simulink library "ServosLib"  (R2022b)
settings: Solver=VariableStepAuto  StartTime=0.0  StopTime=10.0  RelTol=1e-3
undefined symbols (not defined in the file): POS_hi, POS_lo, SimPar
libraries: simulink x2
settings Model: Creator=tbritton  LastModifiedBy=macheson
settings SolverCC: AlgebraicLoopSolver=TrustRegion
settings DebuggingCC: UnconnectedInputMsg=warning  UnconnectedOutputMsg=warning  UnconnectedLineMsg=warning  SFMachineParentedDataDiag=warning
settings ModelReferenceCC: EnableRefExpFcnMdlSchedulingChecks=on
settings RTWCC: DLArmComputeVersion=19.05

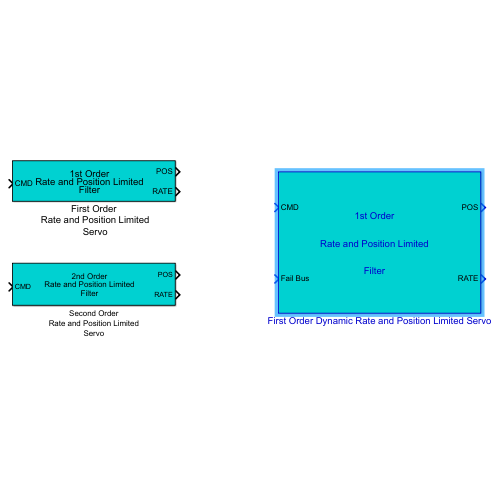
[thumbnail: Simulink's stored preview of the top-level diagram]
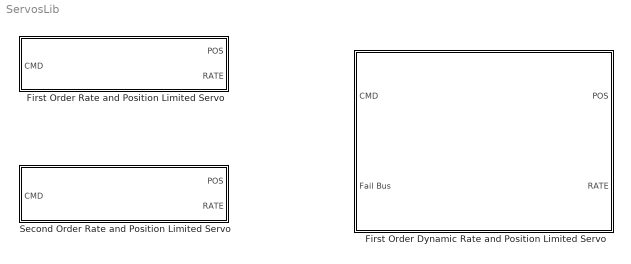
== system ServosLib ==
  First Order Rate and Position Limited Servo : Subsystem  mask(Rate and Position Limited Servo){freq=5, RL=300, POS_hi=30*pi/180, POS_lo=0*pi/180, Bias=0*pi/180, StateName=Actuators}
      mask prompts: freq "Bandwidth, Hz:"; RL "Rate Limit, rad/s:"; POS_hi "Position Limit High, rad:"; POS_lo "Position Limit Low, rad:"; Bias "Bias Value, rad:"; StateName "State Name:"
      mask help: First order transfer function: w/(s+w), with rate and position limits and output bias level.
      mask init:
      | %omega=2*pi*freq;
      mask Display:
      | text(.48,.70,'1st Order','horizontalAlignment','center');
      | text(.48,.50,'Rate and Position Limited','horizontalAlignment','center');
      | text(.48,.30,'Filter','horizontalAlignment','center');
  First Order Dynamic Rate and Position Limited Servo : Subsystem  mask(Rate and Position Limited Servo){freq=SimPar.Actuator.BW, Bias=SimPar.Actuator.Bias, StateName='Actuators'}
      mask prompts: freq "Bandwidth, Hz:"; Bias "Bias Value, rad:"; StateName "State Name:"
      mask help: First order transfer function: w/(s+w), with rate and position limits and output bias level.
      mask init:
      | %omega=2*pi*freq;
      mask Display:
      | text(.48,.70,'1st Order','horizontalAlignment','center');
      | text(.48,.50,'Rate and Position Limited','horizontalAlignment','center');
      | text(.48,.30,'Filter','horizontalAlignment','center');
  Second Order Rate and Position Limited Servo : Subsystem  mask(Rate and Position Limited Servo){freq=5, zeta=0.7, RL=300, POS_hi=30*pi/180, POS_lo=0*pi/180, Bias=0*pi/180, PosStateName=ActuatorPosition, RateStateName=ActuatorRate}
      mask prompts: freq "Bandwidth, Hz:"; zeta "Damping Ratio:"; RL "Rate Limit, rad/s:"; POS_hi "Position Limit High, rad:"; POS_lo "Position Limit Low, rad:"; Bias "Bias Value, rad:"; PosStateName "Position State Name:"; RateStateName "Rate State Name:"
      mask help: Second order transfer function: w^2/(s^2+2*zeta*w*s+w^2), with rate and position limits and output bias level.
      mask init:
      | %omega=2*pi*freq;
      mask Display:
      | text(.48,.70,'2nd Order','horizontalAlignment','center');
      | text(.48,.50,'Rate and Position Limited','horizontalAlignment','center');
      | text(.48,.30,'Filter','horizontalAlignment','center');

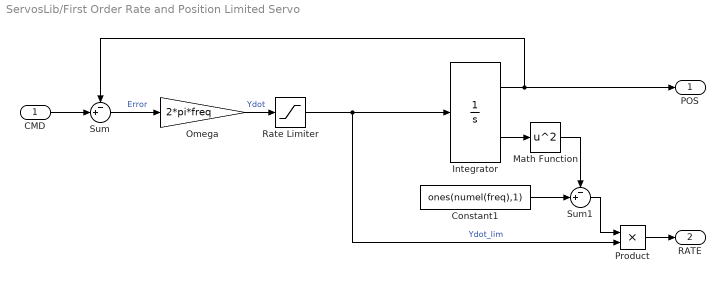
== system ServosLib/First Order Rate and Position Limited Servo ==
  CMD : Inport
  Constant1 : Constant  Value=ones(numel(freq),1)  VectorParams1D=off
  Integrator : Integrator  InitialCondition=Bias  LimitOutput=on  UpperSaturationLimit=POS_hi  LowerSaturationLimit=POS_lo  ShowSaturationPort=on  IgnoreLimit=on  ContinuousStateAttributes=StateName
  Math Function : Math  Operator=square  SignedPower=on
  Omega : Gain  Gain=2*pi*freq  SaturateOnIntegerOverflow=on  OutDataTypeStr=Inherit: Same as input  ParamDataTypeStr=Inherit: Same as input
  Product : Product  RndMeth=Zero
  Rate Limiter : Saturate  UpperLimit=RL  LowerLimit=-RL
  Sum : Sum  Inputs=-+|  InputSameDT=on  SaturateOnIntegerOverflow=on  OutDataTypeStr=Inherit: Same as first input
  Sum1 : Sum  Inputs=-+|  InputSameDT=on  SaturateOnIntegerOverflow=on  OutDataTypeStr=Inherit: Same as first input
  POS : Outport  VectorParamsAs1DForOutWhenUnconnected=off
  RATE : Outport  Port=2
  wires:
  CMD/1 -> Sum/2
  Rate Limiter/1 -> Integrator/1, Product/2  "Ydot_lim"
  Integrator/1 -> POS/1, Sum/1
  Sum/1 -> Omega/1  "Error"
  Omega/1 -> Rate Limiter/1  "Ydot"
  Integrator/2 -> Math Function/1
  Sum1/1 -> Product/1
  Product/1 -> RATE/1
  Constant1/1 -> Sum1/2
  Math Function/1 -> Sum1/1

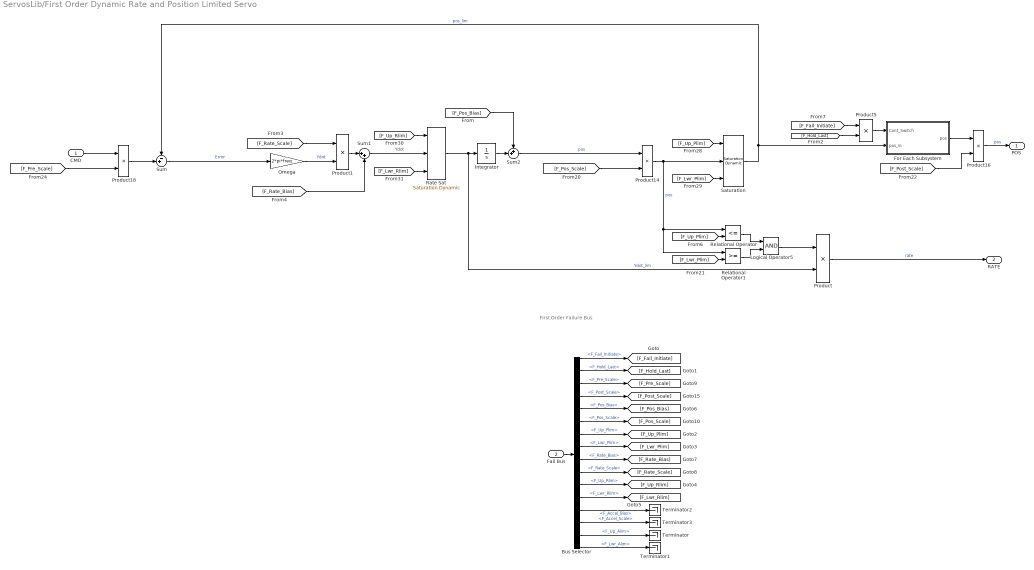
== system ServosLib/First Order Dynamic Rate and Position Limited Servo ==
  note: First Order Failure Bus
  CMD : Inport
  Fail Bus : Inport  Port=2
  Bus Selector : BusSelector  OutputSignals=F_Fail_Initiate,F_Hold_Last,F_Pre_Scale,F_Post_Scale,F_Pos_Bias,F_Pos_Scale,F_Up_Plim,F_Lwr_Plim,F_Rate_Bias,F_Rate_Scale,F_Up_Rlim,F_Lwr_Rlim,F_Accel_Bias,F_Accel_Scale,F_Up_Alim,F_Lwr_Alim
  For Each Subsystem : Subsystem  TreatAsAtomicUnit=on
  Integrator : Integrator  InitialCondition=Bias  UpperSaturationLimit=POS_hi  LowerSaturationLimit=POS_lo  IgnoreLimit=on  ContinuousStateAttributes=StateName
  Logical Operator5 : Logic  AllPortsSameDT=off  OutDataTypeStr=boolean
  Omega : Gain  Gain=2*pi*freq  SaturateOnIntegerOverflow=on  OutDataTypeStr=Inherit: Same as input  ParamDataTypeStr=Inherit: Same as input
  Product : Product  RndMeth=Zero
  Product{1,5,14,16,18} (5 alike) : Product
  Rate Sat : simulink/Discontinuities/Saturation Dynamic  OutMin=[]  OutMax=[]  OutDataTypeStr=Inherit: Same as second input  OutDataType=fixdt(1, 16)  OutScaling=2^-10  DoSatur=off
  Relational Operator : RelationalOperator  Operator=<=  OutDataTypeStr=boolean  RndMeth=Simplest  InputSameDT=off
  Relational Operator1 : RelationalOperator  OutDataTypeStr=boolean  RndMeth=Simplest  InputSameDT=off
  Saturation : simulink/Discontinuities/Saturation Dynamic  OutMin=[]  OutMax=[]  OutDataTypeStr=Inherit: Same as second input  OutDataType=fixdt(1, 16)  OutScaling=2^-10  DoSatur=off
  Sum : Sum  Inputs=-+|  InputSameDT=on  SaturateOnIntegerOverflow=on  OutDataTypeStr=Inherit: Same as first input
  Sum1 : Sum  Inputs=|++  InputSameDT=on  SaturateOnIntegerOverflow=on  OutDataTypeStr=Inherit: Same as first input
  Sum2 : Sum  Inputs=++|
  Terminator{,1..3} (4 alike) : Terminator
  POS : Outport  VectorParamsAs1DForOutWhenUnconnected=off
  RATE : Outport  Port=2
  wires:
  CMD/1 -> Product18/1
  Rate Sat/1 -> Product/2, Integrator/1  "Ydot_lim"
  Sum/1 -> Omega/1  "Error"
  Omega/1 -> Product1/2  "Ydot"
  Product/1 -> RATE/1  "rate"
  Fail Bus/1 -> Bus Selector/1
  Bus Selector/1 -> [F_Fail_Initiate]  "<F_Fail_Initiate>"
  Bus Selector/2 -> [F_Hold_Last]  "<F_Hold_Last>"
  Product14/1 -> Relational Operator1/1, Relational Operator/1, Saturation/2  "pos"
  Saturation/1 -> For Each Subsystem/2(pos_in), Sum/1  "pos_lim"
  Integrator/1 -> Sum2/2
  [F_Hold_Last] -> Product5/2
  For Each Subsystem/1(pos) -> Product16/1
  Sum1/1 -> Rate Sat/2  "Ydot"
  Product1/1 -> Sum1/1
  Bus Selector/5 -> [F_Pos_Bias]  "<F_Pos_Bias>"
  Bus Selector/10 -> [F_Rate_Scale]  "<F_Rate_Scale>"
  Bus Selector/9 -> [F_Rate_Bias]  "<F_Rate_Bias>"
  Bus Selector/13 -> Terminator2/1  "<F_Accel_Bias>"
  Bus Selector/14 -> Terminator3/1  "<F_Accel_Scale>"
  Product5/1 -> For Each Subsystem/1(Cont_Switch)
  [F_Fail_Initiate] -> Product5/1
  Bus Selector/15 -> Terminator/1  "<F_Up_Alim>"
  Bus Selector/16 -> Terminator1/1  "<F_Lwr_Alim>"
  Bus Selector/7 -> [F_Up_Plim]  "<F_Up_Plim>"
  Bus Selector/8 -> [F_Lwr_Plim]  "<F_Lwr_Plim>"
  Bus Selector/11 -> [F_Up_Rlim]  "<F_Up_Rlim>"
  Bus Selector/12 -> [F_Lwr_Rlim]  "<F_Lwr_Rlim>"
  [F_Up_Rlim] -> Rate Sat/1
  [F_Lwr_Rlim] -> Rate Sat/3
  [F_Up_Plim] -> Saturation/1
  [F_Lwr_Plim] -> Saturation/3
  Sum2/1 -> Product14/1  "pos"
  Bus Selector/6 -> [F_Pos_Scale]  "<F_Pos_Scale>"
  [F_Post_Scale] -> Product16/2
  Product16/1 -> POS/1  "pos"
  [F_Pre_Scale] -> Product18/2
  Product18/1 -> Sum/2
  Bus Selector/4 -> [F_Post_Scale]  "<F_Post_Scale>"
  Bus Selector/3 -> [F_Pre_Scale]  "<F_Pre_Scale>"
  [F_Rate_Bias] -> Sum1/2
  [F_Rate_Scale] -> Product1/1
  [F_Pos_Bias] -> Sum2/1
  [F_Pos_Scale] -> Product14/2
  [F_Up_Plim] -> Relational Operator/2
  [F_Lwr_Plim] -> Relational Operator1/2
  Relational Operator/1 -> Logical Operator5/1
  Relational Operator1/1 -> Logical Operator5/2
  Logical Operator5/1 -> Product/1

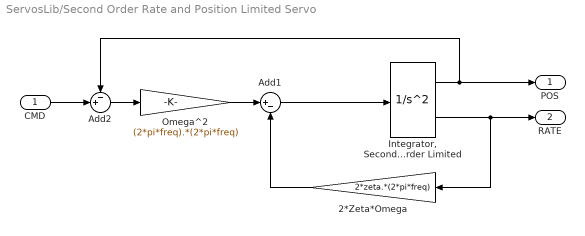
== system ServosLib/Second Order Rate and Position Limited Servo ==
  CMD : Inport
  2*Zeta*Omega : Gain  Gain=2*zeta.*(2*pi*freq)
  Add1 : Sum  Inputs=|+-
  Add2 : Sum  Inputs=-+|
  "Integrator, Second-Order Limited" : SecondOrderIntegrator  ICX=Bias  LimitX=on  UpperLimitX=POS_hi  LowerLimitX=POS_lo  StateNameX=PosStateName  LimitDXDT=on  UpperLimitDXDT=RL  LowerLimitDXDT=-RL  StateNameDXDT=RateStateName  IgnoreStateLimitsAndResetForLinearization=on
  Omega^2 : Gain  Gain=(2*pi*freq).*(2*pi*freq)
  POS : Outport
  RATE : Outport  Port=2
  wires:
  CMD/1 -> Add2/2
  "Integrator, Second-Order Limited"/2 -> RATE/1, 2*Zeta*Omega/1
  Omega^2/1 -> Add1/1
  Add2/1 -> Omega^2/1
  "Integrator, Second-Order Limited"/1 -> POS/1, Add2/1
  2*Zeta*Omega/1 -> Add1/2
  Add1/1 -> "Integrator, Second-Order Limited"/1

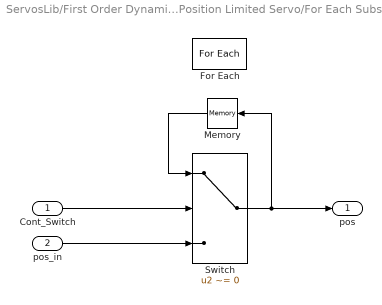
== system ServosLib/First Order Dynamic Rate and Position Limited Servo/For Each Subsystem ==
  Cont_Switch : Inport  Partition=on  PartitionDimension=1  PartitionWidth=1  PartitionOffset=0
  pos_in : Inport  Port=2  Partition=on  PartitionDimension=1  PartitionWidth=1  PartitionOffset=0
  For Each : ForEach  DisableCoverage=on
  Memory : Memory
  Switch : Switch  Criteria=u2 ~= 0  SaturateOnIntegerOverflow=off  InputSameDT=off
  pos : Outport  ConcatenationDimension=1
  wires:
  pos_in/1 -> Switch/3
  Cont_Switch/1 -> Switch/2
  Switch/1 -> pos/1, Memory/1
  Memory/1 -> Switch/1
